simulink model "simpleModel_lstm"  (R2023a)
settings: Solver=FixedStepAuto  StartTime=0.0  StopTime=10.0  FixedStep=0.01  RelTol=1e-3
libraries: SignalEditorBlockLib x1, deeplib x1
settings Model: Creator=imyrsini  LastModifiedBy=imyrsini

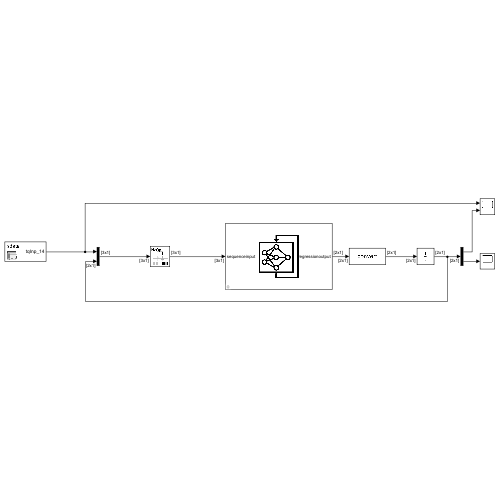
[thumbnail: Simulink's stored preview of the top-level diagram]
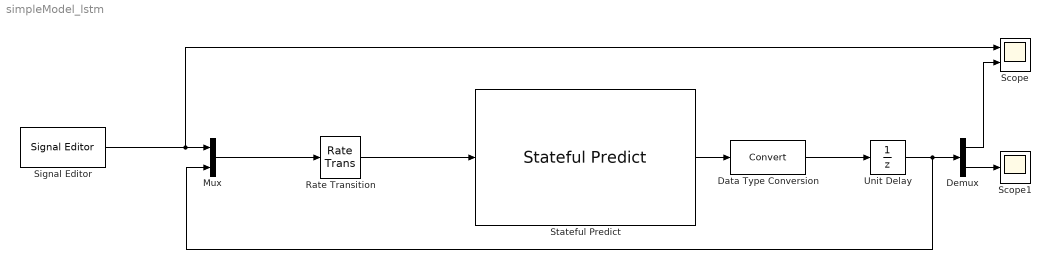
== system simpleModel_lstm ==
  Data Type Conversion : DataTypeConversion  SaturateOnIntegerOverflow=off  RndMeth=Floor
  Demux : Demux  Outputs=2
  Mux : Mux  Inputs=2
  Rate Transition : RateTransition  OutPortSampleTime=0.01
  Scope : Scope  NumInputPorts=2
  Scope1 : Scope
  Signal Editor : SignalEditorBlockLib/Signal Editor  FileName=tqInp_14.mat  ActiveScenario=sdata  ActiveSignal=tqInp_14  IsBus=off  OutputBusObjectStr=Bus: BusObject  SampleTime=0  Interpolate=off  ZeroCross=off  OutputAfterFinalValue=Setting to zero  Unit=inherit  PreserveSignalName=on  ApplySigPropsToAllScenarios=on
  Stateful Predict : deeplib/Stateful Predict  Network=Network from MAT-file  NetworkFunction=untitled  NetworkFilePath=C:\Users\imyrsini\OneDrive - MathWorks\Documents\Projects\AEprojects\LSTM Model Reduction\netExp1.mat  InputDataFormats={'',''}  SampleTime=-1  ForceInterpretedSim=off  EnableDLNetwork=on
  Unit Delay : UnitDelay  InitialCondition=[0; 0]  SampleTime=-1  HasFrameUpgradeWarning=on
  wires:
  Unit Delay/1 -> Demux/1, Mux/2
  Data Type Conversion/1 -> Unit Delay/1
  Rate Transition/1 -> Stateful Predict/1
  Stateful Predict/1 -> Data Type Conversion/1
  Signal Editor/1 -> Scope/1, Mux/1
  Mux/1 -> Rate Transition/1
  Demux/1 -> Scope/2
  Demux/2 -> Scope1/1
